simulink model "adap_filt"  (R2020b)
settings: Solver=VariableStepAuto  StartTime=0.0  StopTime=10.0  MaxStep=0.00001  RelTol=1e-3
settings Model: Creator=akif  LastModifiedBy=akif

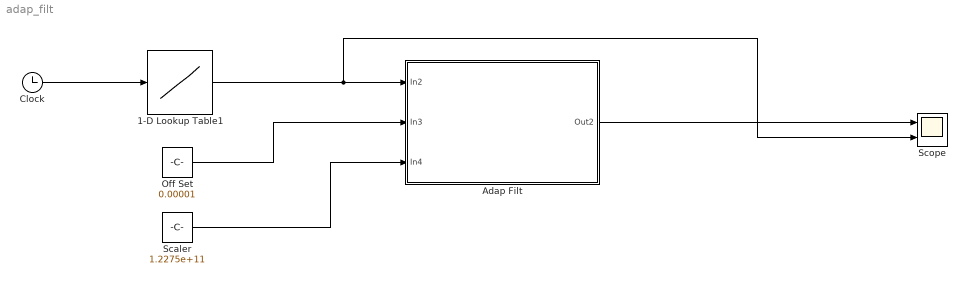
== system adap_filt ==
  1-D Lookup Table1 : Lookup_n-D  NumberOfTableDimensions=1  BreakpointsForDimension1=[1:316]/316*10  Table=|  InternalRulePriority=Speed  RndMeth=Simplest  InputSameDT=on
      | [1.64051362843654e-05
      | 1.40568629590453e-05
      | 2.38051839122959e-05
      | 8.74148729451735e-06
      | 1.06554794518674e-05
      | 9.42977118655720e-06
      | 6.32057670890317e-06
      | 9.01997895240314e-06
      | 1.49954346164976e-05
      | 9.58231596614020e-06
      | 7.50980209858022e-06
      | 1.59194850623294e-05
      | 1.76468436451053e-05
      | 1.45851301015796e-05
      | 1.15162942135961e-05
      | 3.04743612052389e-05
      | 2.05245951273964e-05
      | 2.06062407375594e-05
      | 1.35867386817611e-05
      | 1.49109876143719e-05
      | 1.43568232486710e-05
      | 1.21885674523159e-05
      | 1.43850622871426e-05
      | 1.30287648769615e-05
      | 1.32877050840663e-05
      | 1.60527488396966e-05
      | 1.31786557673880e-05
      | 1.69549726504939e-05
      | 1.16456487503651e-05
      | 2.05296487816749e-05
      | 1.22177852958360e-05
      | 2.16842945376947e-05
      | 1.69746251737210e-05
      | 1.81593586811865e-05
      | 1.37955055880923e-05
      | 1.18149305849060e-05
      | 1.80562629304544e-05
      | 2.00360706115520e-05
      | 1.65161466091022e-05
      | 1.42931315618229e-05
      | 1.26379536135817e-05
      | 9.37777273375010e-06
      | 2.50012715700335e-05
      | 9.80946252505066e-06
      | 1.25063878950349e-05
      | 1.54944614887166e-05
      | 1.86334828135967e-05
      | 2.67535074162875e-05
      | 2.17668938779652e-05
      | 1.57583560398039e-05
      | 1.62689315481486e-05
      | 2.57638329268482e-05
      | 2.41916142849367e-05
      | 1.50075467750277e-05
      | 1.48414296964411e-05
      | 1.85642687658673e-05
      | 1.86472801850234e-05
      | 1.40826481782088e-05
      | 1.82000138000706e-05
      | 2.33472369265069e-05
      | 1.65835079337188e-05
      | 1.67766145979206e-05
      | 1.76127493793897e-05
      | 9.83805933311541e-06
      | 1.74140156542087e-05
      | 1.50925179008052e-05
      | 1.80161561234154e-05
      | 1.79132967525853e-05
      | 1.00795451975540e-05
      | 1.85132815783139e-05
      | 1.28150943354413e-05
      | 1.25145964319652e-05
      | 2.03877350233099e-05
      | 2.09833224887680e-05
      | 1.58582483478149e-05
      | 2.30398667189581e-05
      | 1.25043660595919e-05
      | 1.32910905088036e-05
      | 2.16697387803888e-05
      | 6.03255120916314e-05
      | 2.25779997098017e-05
      | 2.45620639329186e-05
      | 1.29174264321843e-05
      | 3.21544263599091e-05
      | 1.70163337381476e-05
      | 1.81629313963242e-05
      | 2.97077939108279e-05
      | 2.10626563633244e-05
      | 1.98639370628822e-05
      | 2.20207256722340e-05
      | 2.13388929195934e-05
      | 1.42943415424987e-05
      | 2.43752771911017e-05
      | 3.29048664796179e-05
      | 2.16699759721797e-05
      | 1.63278058873523e-05
      | 2.27822590013486e-05
      | 1.02346038265266e-05
      | 1.85384983866811e-05
      | 2.37260916269941e-05
      | 1.40450116446675e-05
      | 1.77256607872559e-05
      | 2.42393091730105e-05
      | 1.77661694819919e-05
      | 1.79875144098504e-05
      | 1.55901254065795e-05
      | 2.29764635856900e-05
      | 1.88738946830650e-05
      | 1.96300738101188e-05
      | 1.22818500124545e-05
      | 1.66247661350135e-05
      | 4.31410092205206e-05
      | 1.90779039880144e-05
      | 2.37161254355536e-05
      | 1.05865490301614e-05
      | 2.30617935321578e-05
      | 2.36026955756572e-05
      | 4.14747699704217e-05
      | 2.92279297682836e-05
      | 2.48898588978181e-05
      | 1.72361854986676e-05
      | 2.69208000199753e-05
      | 2.43689611029871e-05
      | 2.72982996626707e-05
      | 1.10285198984475e-05
      | 2.47721145476778e-05
      | 1.89354625232408e-05
      | 3.02766165777375e-05
      | 1.96450536145204e-05
      | 1.39331476140752e-05
      | 2.02457718492409e-05
      | 1.22273270980727e-05
      | 2.87292582767595e-05
      | 2.46312159117051e-05
      | 1.40335194655741e-05
      | 2.96224263762219e-05
      | 1.34466083600585e-05
      | 2.15909899463688e-05
      | 1.41221455064165e-05
      | 3.19288484839238e-05
      | 1.86219373721577e-05
      | 1.74748422158834e-05
      | 1.09792145249926e-05
      | 7.27746946998597e-05
      | 2.90071508924096e-05
      | 2.81134943505450e-05
      | 3.45389338471732e-05
      | 2.12919130338529e-05
      | 1.61115007349485e-05
      | 2.08763034476168e-05
      | 1.08860514380027e-05
      | 1.79059951043661e-05
      | 2.17391005942320e-05
      | 1.36301674336495e-05
      | 2.23018266116876e-05
      | 2.33487228977312e-05
      | 2.00897504932878e-05
      | 3.08220860199014e-05
      | 1.89658071937624e-05
      | 1.39060025495346e-05
      | 1.80894795685976e-05
      | 1.91431356481945e-05
      | 4.47639205320871e-05
      | 4.06901736875501e-05
      | 2.38466380703158e-05
      | 2.11172112389638e-05
      | 1.88146295524957e-05
      | 1.15677485667651e-05
      | 1.46668996322195e-05
      | 2.34706427416889e-05
      | 1.22777034103040e-05
      | 2.52989639512073e-05
      | 2.23519705472901e-05
      | 2.46894725889954e-05
      | 2.67729206265021e-05
      | 4.22178959395528e-05
      | 2.16833323682248e-05
      | 1.57552372239104e-05
      | 1.52405921937705e-05
      | 1.53498025872232e-05
      | 2.22961900295201e-05
      | 1.78825933483340e-05
      | 2.41598236604577e-05
      | 1.64931904337819e-05
      | 2.14074897132851e-05
      | 1.75742564379662e-05
      | 2.34699558591484e-05
      | 1.77773758697096e-05
      | 2.12706595995984e-05
      | 1.72275320129192e-05
      | 2.01383973493276e-05
      | 2.34672366895503e-05
      | 2.28803316634854e-05
      | 2.16461798602177e-05
      | 2.07837136999138e-05
      | 1.80824126660207e-05
      | 3.49555691729447e-05
      | 2.78864031885556e-05
      | 1.93679648743161e-05
      | 1.15901945645408e-05
      | 1.82902148658386e-05
      | 2.03209236064996e-05
      | 3.36660271174276e-05
      | 2.71618502199090e-05
      | 2.49204310646066e-05
      | 2.90768019108371e-05
      | 2.51928543513350e-05
      | 9.67134026027886e-05
      | 3.38920244691419e-05
      | 3.06693919201756e-05
      | 1.76453388658974e-05
      | 2.18975284435949e-05
      | 2.10859871673180e-05
      | 1.71801565079614e-05
      | 2.82088936242430e-05
      | 2.35496220830208e-05
      | 2.83451960308777e-05
      | 2.29397033642108e-05
      | 2.00922272431655e-05
      | 2.46108276739707e-05
      | 2.08911355590200e-05
      | 2.31728752078192e-05
      | 1.45757663135255e-05
      | 1.81867614869434e-05
      | 1.98370079026519e-05
      | 3.38130774632942e-05
      | 2.57446660399387e-05
      | 1.88870716654182e-05
      | 2.07980739595268e-05
      | 1.63812752458330e-05
      | 3.80699989099892e-05
      | 2.40169859437470e-05
      | 1.33996635493158e-05
      | 1.57553699372538e-05
      | 9.61083642856393e-06
      | 1.86813680959446e-05
      | 1.95015552404810e-05
      | 1.21563499912564e-05
      | 1.43772284824941e-05
      | 5.30010206166962e-05
      | 2.58550539438812e-05
      | 3.41669985603186e-05
      | 2.54261518011405e-05
      | 1.38597890554647e-05
      | 1.93920388086061e-05
      | 1.71392873719934e-05
      | 2.44790490913431e-05
      | 2.50734812581297e-05
      | 2.34272211045535e-05
      | 2.12306279716383e-05
      | 1.30868829754710e-05
      | 1.78155321907224e-05
      | 2.83193727687242e-05
      | 3.03118667377854e-05
      | 1.59936839959617e-05
      | 3.34627690473215e-05
      | 2.08213213025020e-05
      | 1.29448749909497e-05
      | 3.10665603094219e-05
      | 3.62883168299117e-05
      | 1.75189510354820e-05
      | 1.60519412140470e-05
      | 2.24211867708450e-05
      | 1.98503234825196e-05
      | 4.07945778967437e-05
      | 4.05952014733018e-05
      | 1.34548331739826e-05
      | 2.01382644046719e-05
      | 2.53975081805474e-05
      | 1.62746865089044e-05
      | 1.98107453316660e-05
      | 7.89869048822377e-05
      | 4.89737997106953e-05
      | 2.40563563126007e-05
      | 2.19373471901125e-05
      | 2.50900186675382e-05
      | 2.57129806994504e-05
      | 1.85411271741837e-05
      | 2.94006448101928e-05
      | 2.83748261733353e-05
      | 2.67237388712814e-05
      | 2.45675583591609e-05
      | 1.49475822704207e-05
      | 2.00668626728808e-05
      | 1.97978678956109e-05
      | 2.54242571517436e-05
      | 1.73245472466924e-05
      | 3.90006558368019e-05
      | 3.28673126709357e-05
      | 3.23222858714683e-05
      | 2.61864572240293e-05
      | 1.92837345867870e-05
      | 2.82020427335874e-05
      | 2.04865733463850e-05
      | 1.72301801766338e-05
      | 5.74247999782434e-05
      | 6.11199214144019e-05
      | 3.44921244452841e-05
      | 3.99599983815840e-05
      | 2.87352773373638e-05
      | 2.63111420997852e-05
      | 1.66206206696214e-05
      | 2.18048961463832e-05
      | 4.62724796986172e-05
      | 2.74893275945451e-05
      | 3.57663192938257e-05
      | 4.56687458805537e-05
      | 2.06372788255615e-05
      | 2.65724334222749e-05
      | 4.06305334690050e-05
      | 3.31941887703738e-05
      | 3.43056023600827e-05
      | 3.58793683642042e-05
      | 1.99642919124117e-05
      | 2.85717950537800e-05
      | 1.42437487415731e-05]
  Adap Filt : Subsystem
  Clock : Clock
  Off Set : Constant  Value=0.00001
  Scaler : Constant  Value=1.2275e+11
  Scope : Scope  NumInputPorts=2
  wires:
  Clock/1 -> 1-D Lookup Table1/1
  1-D Lookup Table1/1 -> Scope/2, Adap Filt/1(In2)
  Off Set/1 -> Adap Filt/2(In3)
  Scaler/1 -> Adap Filt/3(In4)
  Adap Filt/1(Out2) -> Scope/1

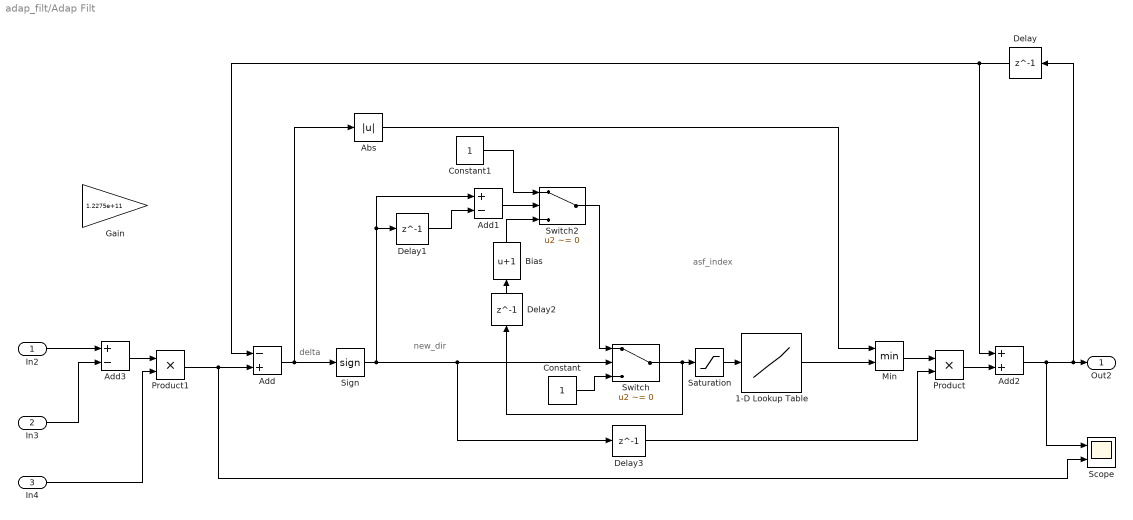
== system adap_filt/Adap Filt ==
  note: delta
  note: asf_index
  note: new_dir
  In2 : Inport
  In3 : Inport  Port=2
  In4 : Inport  Port=3
  1-D Lookup Table : Lookup_n-D  NumberOfTableDimensions=1  BreakpointsForDimension1=[1: 25]  Table=[1,1,1,1,2,2,2,2,2,3,3,3,3,4,4,5,5,6,7,8,9,9,10,11,11]  InternalRulePriority=Speed  RndMeth=Simplest  InputSameDT=on
  Abs : Abs
  Add : Sum  Inputs=-+
  Add1 : Sum  Inputs=+-
  Add2 : Sum
  Add3 : Sum  Inputs=+-
  Bias : Bias  Bias=1
  Constant : Constant
  Constant1 : Constant
  Delay{,1..3} (4 alike) : Delay  DelayLength=1
  Gain : Gain  Gain=1.2275e+11
  Min : MinMax  Inputs=2
  Product : Product
  Product1 : Product
  Saturation : Saturate  UpperLimit=25  LowerLimit=1
  Scope : Scope  NumInputPorts=2
  Sign : Signum
  Switch : Switch  Criteria=u2 ~= 0
  Switch2 : Switch  Criteria=u2 ~= 0
  Out2 : Outport
  wires:
  In2/1 -> Add3/1
  In4/1 -> Product1/2
  Add3/1 -> Product1/1
  Saturation/1 -> 1-D Lookup Table/1
  Constant/1 -> Switch/3
  Switch/1 -> Delay2/1, Saturation/1
  In3/1 -> Add3/2
  Delay2/1 -> Bias/1
  Product1/1 -> Scope/2, Add/2
  Delay/1 -> Add2/1, Add/1
  Bias/1 -> Switch2/3
  Add/1 -> Abs/1, Sign/1
  Add1/1 -> Switch2/2
  Sign/1 -> Add1/1, Delay1/1, Delay3/1, Switch/2
  Delay1/1 -> Add1/2
  Constant1/1 -> Switch2/1
  Add2/1 -> Delay/1, Out2/1, Scope/1
  Product/1 -> Add2/2
  Switch2/1 -> Switch/1
  Min/1 -> Product/1
  Delay3/1 -> Product/2
  1-D Lookup Table/1 -> Min/2
  Abs/1 -> Min/1
